simulink model "dynamicsquat"  (R2023a)
settings: Solver=VariableStepAuto  StartTime=0.0  StopTime=stoptimetotal  RelTol=1e-3
values from neighbouring files (symbols this model uses):
  battery = load('params/battery_Tattu.mat').battery    [runDetailedT18Model.m]
  IC = load('params/initialcond/IC_HoverAt30mOcto.mat').IC    [runDetailedT18Model.m]
  maxleashvelocity = 5    [runDetailedT18Model.m]
  Motor = load('params/KDE4213XF-360_performancedata.mat').Motor    [runDetailedT18Model.m]
  octomodel = load('params/TarotT18.mat').octomodel    [runDetailedT18Model.m]
  turbenabled = 0    [runDetailedT18Model.m]
  xref = xyzref(waypts,1)    [runDetailedT18Model.m]
  yref = xyzref(waypts,2)    [runDetailedT18Model.m]
  zref = xyzref(waypts,3)    [runDetailedT18Model.m]
undefined symbols (not defined in the file or in its folder): deg, DiscIntNeverNeededParam, F, Light, MIL, rad, s
libraries: aerolibconvert2 x2, shared6dof x1, aerolibwind2 x1
(part 2 of 2)

== system dynamicsquat/Motors/DC Motor 3/Mechanical part/torque and thrust calculation ==
  w angular speed : Inport
  Convert rad/s to rmp : Gain  Gain=60/(2*pi)
  "Propeller model " : MATLAB Function  TreatAsAtomicUnit=on
  torque : Outport  VectorParamsAs1DForOutWhenUnconnected=off
  thrusth : Outport  Port=2  VectorParamsAs1DForOutWhenUnconnected=off
  wires:
  Convert rad/s to rmp/1 -> "Propeller model "/1(rpm)
  w angular speed/1 -> Convert rad/s to rmp/1
  "Propeller model "/2(thrust) -> thrusth/1
  "Propeller model "/1(torque) -> torque/1

== system dynamicsquat/Motors/DC Motor 4/Mechanical part/torque and thrust calculation ==
  w angular speed : Inport
  Convert rad/s to rmp : Gain  Gain=60/(2*pi)
  "Propeller model " : MATLAB Function  TreatAsAtomicUnit=on
  torque : Outport  VectorParamsAs1DForOutWhenUnconnected=off
  thrusth : Outport  Port=2  VectorParamsAs1DForOutWhenUnconnected=off
  wires:
  "Propeller model "/1(torque) -> torque/1
  "Propeller model "/2(thrust) -> thrusth/1
  w angular speed/1 -> Convert rad/s to rmp/1
  Convert rad/s to rmp/1 -> "Propeller model "/1(rpm)

== system dynamicsquat/Motors/DC Motor 5/Mechanical part/torque and thrust calculation ==
  w angular speed : Inport
  Convert rad/s to rmp : Gain  Gain=60/(2*pi)
  "Propeller model " : MATLAB Function  TreatAsAtomicUnit=on
  torque : Outport  VectorParamsAs1DForOutWhenUnconnected=off
  thrusth : Outport  Port=2  VectorParamsAs1DForOutWhenUnconnected=off
  wires:
  Convert rad/s to rmp/1 -> "Propeller model "/1(rpm)
  w angular speed/1 -> Convert rad/s to rmp/1
  "Propeller model "/2(thrust) -> thrusth/1
  "Propeller model "/1(torque) -> torque/1

== system dynamicsquat/Motors/DC Motor 6/Mechanical part/torque and thrust calculation ==
  w angular speed : Inport
  Convert rad/s to rmp : Gain  Gain=60/(2*pi)
  "Propeller model " : MATLAB Function  TreatAsAtomicUnit=on
  torque : Outport  VectorParamsAs1DForOutWhenUnconnected=off
  thrusth : Outport  Port=2  VectorParamsAs1DForOutWhenUnconnected=off
  wires:
  "Propeller model "/1(torque) -> torque/1
  "Propeller model "/2(thrust) -> thrusth/1
  w angular speed/1 -> Convert rad/s to rmp/1
  Convert rad/s to rmp/1 -> "Propeller model "/1(rpm)

== system dynamicsquat/Motors/DC Motor 7/Mechanical part/torque and thrust calculation ==
  w angular speed : Inport
  Convert rad/s to rmp : Gain  Gain=60/(2*pi)
  "Propeller model " : MATLAB Function  TreatAsAtomicUnit=on
  torque : Outport  VectorParamsAs1DForOutWhenUnconnected=off
  thrusth : Outport  Port=2  VectorParamsAs1DForOutWhenUnconnected=off
  wires:
  Convert rad/s to rmp/1 -> "Propeller model "/1(rpm)
  w angular speed/1 -> Convert rad/s to rmp/1
  "Propeller model "/2(thrust) -> thrusth/1
  "Propeller model "/1(torque) -> torque/1

== system dynamicsquat/Motors/DC Motor 8/Mechanical part/torque and thrust calculation ==
  w angular speed : Inport
  Convert rad/s to rmp : Gain  Gain=60/(2*pi)
  "Propeller model " : MATLAB Function  TreatAsAtomicUnit=on
  torque : Outport  VectorParamsAs1DForOutWhenUnconnected=off
  thrusth : Outport  Port=2  VectorParamsAs1DForOutWhenUnconnected=off
  wires:
  "Propeller model "/1(torque) -> torque/1
  "Propeller model "/2(thrust) -> thrusth/1
  w angular speed/1 -> Convert rad/s to rmp/1
  Convert rad/s to rmp/1 -> "Propeller model "/1(rpm)

== matlab function dynamicsquat/Motors/DC Motor 8/Mechanical part/torque and thrust calculation/Propeller model  ==
  data: torque output; rpm input; thrust output
function [torque,thrust] = fcn(rpm)
%% Tarot model data

%coefficient of thrust, empirically derived
coef_t = 0.065;
%thrust = coef_t * density of air * velocity^2 * propeller diameter (m) ^4
%velocity in rev/sec, where  1 rev/sec = 1 rpm/60
thrust = coef_t*1.225*(rpm/60)^2*.47^4; % 18.5 inches ~ 0.47 m
% empirically derived
torque = (2.138e-08)*rpm^2 + (-1.279e-05)*rpm ;% (0.0216);

end

== matlab function dynamicsquat/Position//Velocity controllers/Velocity leashing ==
  data: refvelx input; ref_velx output; refvely input; refvelz input; The input; Phi input; Psi input; max_velocity input; ref_vely output; ref_velz output
function [ref_velx,ref_vely,ref_velz] = fcn(refvelx,refvely,refvelz,The,Phi,Psi,max_velocity)
%% convert to body frame velocity

% Earth/local/inertial to body frame DCM matrix (use transpose to transform to body frame from earth)
R_b_e = [cos(Psi)*cos(The) cos(Psi)*sin(The)*sin(Phi)-sin(Psi)*cos(Phi) cos(Psi)*sin(The)*cos(Phi)+sin(Psi)*sin(Phi);
       sin(Psi)*cos(The) sin(Psi)*sin(The)*sin(Phi)+cos(Psi)*cos(Phi) sin(Psi)*sin(The)*cos(Phi)-cos(Psi)*sin(Phi);
       -sin(The)         cos(The)*sin(Phi)                            cos(The)*cos(Phi)]; 

velinert=[refvelx,refvely,refvelz]';
velbody=R_b_e'*velinert;
velbody(3)=velinert(3);%z velocity measurement follows a different principle thus not affected by Euler angles

%% constraint max velocity 
ref_velocity=zeros(1,3);
if abs(norm(velbody)+ 1e-6)>max_velocity
    % preserve direction but constraint total velocity to max
    ref_velocity=(velbody/(norm(velbody)+ 1e-6))* max_velocity;
else
    ref_velocity=velbody;
end

 ref_velx=ref_velocity(1);
 ref_vely=ref_velocity(2);  
 ref_velz=ref_velocity(3);

== matlab function dynamicsquat/Power Consumption Calculation ==
  data: DC input; tot_mot_i output; Imot input
function tot_mot_i  = fcn(DC,Imot)
imot=zeros(8,1);
for i=1:length(DC)
    imot(i)=DC(i)*Imot(i);
end
tot_mot_i=sum(imot);
tot_mot_i=sum(Imot);
end

== matlab function dynamicsquat/Drag Force and Moment Calculation ==
  data: Vw_nom input; Fdrag output; Vw_turb input; Vb input; wb input; Mdrag output; Eul input; windspecs parameter
function [Fdrag,Mdrag]  = fcn(Vw_nom,Vw_turb,Vb,wb,Eul, windspecs)
%% Parameters 
% windspecs - airframe wind-related specs
% Vw_nom - nominal wind velocity in m/s in inertial frame
% Vw_turb - turbulence wind velocity in m/s in inertial frame
% Vb - linear velocity body frame
% wb - angular velocity body frame
% Eul - Euler angles inertial frame
model = windspecs;

% Z-Y-X rotation convention 
Phi = Eul(1);
The = Eul(2);
Psi = Eul(3);
R_b_e = [cos(Psi)*cos(The) cos(Psi)*sin(The)*sin(Phi)-sin(Psi)*cos(Phi) cos(Psi)*sin(The)*cos(Phi)+sin(Psi)*sin(Phi);
       sin(Psi)*cos(The) sin(Psi)*sin(The)*sin(Phi)+cos(Psi)*cos(Phi) sin(Psi)*sin(The)*cos(Phi)-cos(Psi)*sin(Phi);
       -sin(The)         cos(The)*sin(Phi)                            cos(The)*cos(Phi)]; % Rib
R_e_b = R_b_e'; % Rbi  

% 3-torque created by drag
p = wb(1);
q = wb(2);
r = wb(3);
Mdrag=(((-1/2)*model.rho*model.cd)*[model.Axy*p*abs(p)*model.lx model.Axy*q*abs(q)*model.ly 8*model.Ayz*r*abs(r)*model.lz])';

% Wind in the inertial frame

v_we=Vw_nom+Vw_turb; % wind velocity in m/s in inertial frame
v_wb=R_e_b*v_we; % wind velocity in m/s in body frame
v_a=v_wb+Vb; % apparent velocity resulting from wind and body

% 3-Drag force
Fdrag=(((-1/2)*model.rho*model.cd)*[model.Ayz*v_a(1)*abs(v_a(1)) model.Axz*v_a(2)*abs(v_a(2)) model.Axy*v_a(3)*abs(v_a(3))])';


end

== matlab function dynamicsquat/Adding attitude//ang vel noise ==
  data: u input; y output
function y = fcn(u)

y = zeros(6,1);
attnoisestd=0.0106;
angvelnoisestd=0.; 
% posnoisestd=0; 
% velnoisestd=0;
noiseatt=attnoisestd.*randn(3,1)*0;
noiseangvel=angvelnoisestd.*randn(3,1)*0;
noise=[noiseatt ;noiseangvel];
y = y + u + noise;

== matlab function dynamicsquat/Position//Velocity controllers/Position controllers ==
  data: reference input; ref_velx output double size=1; measurement input; ref_vely output double size=1; ref_velz output; errprev input size=[2 1]; errprev output; time input
function [ref_velx,ref_vely,ref_velz,errprev] = fcn(reference,measurement,errprev,time)
%% parameters
k_p=0.5;
k_d=0.05;%ki=;
dt=0.01; %controller frequency
% radius=2;

%% xyz separation

if time>0.12
    see=3.22;
end

%% z control signal calculation
kz_p=0.4;
errz = reference(3) - measurement(3);

% calculate desired velocity for z axis
err_pz = kz_p * errz; % offset based on minimum thrust to hover
ref_velz=err_pz;

%% xy control signal calculation
err = reference(1:2) - measurement(1:2);

%proximity check
% if abs(err(1))<radius
%     err(1)=0;
% end
% if abs(err(2))<radius
%     err(2)=0;
% end

% calculate desired velocity for xy axis
err_p = k_p * err;
% err_i = self.k_i * np.clip(
%     self.err_i + trapezoid((self.err, err), dx=self.dt, axis=0),
%     a_min=-self.max_err_i, a_max=self.max_err_i
% )
err_d = k_d * (err - errprev) / dt;
%direct velocity usage
ref_velxy=zeros(1,2);
ref_velx = err_p(1) ;%+ err_d2;%+ self.err_i ;
ref_vely = err_p(2) ;%+ err_d2;%+ self.err_i ;

% %% convert total vel to body-frame velocity
% velocity=zeros(1,3);
% velocity=[ref_velxy ref_velz];
% rot = [cos(yaw)   sin(yaw) 0; ...
%     -sin(yaw) cos(yaw) 0; ...
%     0           0      1];
% ref_velocity = rot * velocity; % velocity is a row vector [vx, vy, vz]
% 
% 
% % constraint max velocity 
% if abs(norm(ref_velocity)+ 1e-6)>max_velocity
%     % preserve direction but constraint total velocity to max
%     ref_velocity=(ref_velocity/norm(ref_velocity)+ 1e-6)* max_velocity;
% end
% 
%  ref_velx=ref_velocity(1);
%  ref_vely=ref_velocity(2);  
%  ref_velz=ref_velocity(3);  
% 
% errprev=err;

== matlab function dynamicsquat/arrival condition ==
  data: currentpos input; arrived output; dest input
function arrived = fcn(currentpos,dest)
result=norm(currentpos-dest);
if result<2 % less than one meter from the goal
    arrived=1;
else
    arrived=0;
end

== matlab function dynamicsquat/Adding position//velocity noise ==
  data: u input; y output
function y = fcn(u)

y = zeros(6,1);
posnoisestd=0.6; % 0.75 gives maximum and minimum of +-3 meters, 0.6 is +-2 meters
velnoisestd=0.02; % originally used 0.025
% posnoisestd=0; 
% velnoisestd=0;
noisepos=posnoisestd.*randn(3,1)*0;
noisevel=velnoisestd.*randn(3,1)*0;
noise=[noisepos ;noisevel];
y = y + u + noise;

y=round(y*100)/100;

== matlab function dynamicsquat/MATLAB Function ==
  data: x input; Wx output; y input; Wy output
function [Wx,Wy] = fcn(x,y)
% Interpolate wind speed components at aircraft position
coefs_u = [ 0.00000000e+00  1.61094414e-10 -7.37058611e-03 -1.48809651e-06...
    -3.68089481e-13 -7.95141020e-06  2.10701150e-17  9.01146727e-10...
    1.59724993e-17  6.10108129e-10  7.28957673e-14  8.49416234e-19...
    7.23116917e-13  4.75030720e-19  1.14705027e-12];
intercept_u = 10.362042657397877;

coefs_v = [ 0.00000000e+00 -2.00488263e-10  8.08528198e-03 -7.92842850e-07...
    4.03295347e-13  3.32875723e-06 -1.06781708e-17 -7.96012216e-11...
    -1.33310503e-17 -4.23514366e-09  7.95707308e-14 -4.36936906e-19...
    -5.13247109e-14 -4.72047951e-19 -1.17203841e-12];
intercept_v = 3.69631689881155;
degree = 4;

% Combine xs and ys into a single matrix of shape (n_samples, n_features)
features = [x, y];

    % Calculate the total number of polynomial features including the bias term
    totalFeatures = (degree + 1) * (degree + 2) / 2;
    
    [n_samples, ~] = size(features);
    
    % Preallocate polyFeatures matrix with zeros
    polyFeatures = zeros(n_samples, totalFeatures);
    
    % Fill in the bias (intercept) term
    polyFeatures(:, 1) = ones(n_samples, 1);
    
    % Index to keep track of the current column in polyFeatures
    currentColumn = 2;
    
    % Generate feature combinations and fill in polyFeatures
    for d = 1:degree
        for i = 0:d
            j = d - i;
            newFeature = (features(:,1).^i) .* (features(:,2).^j);
            polyFeatures(:, currentColumn) = newFeature;
            currentColumn = currentColumn + 1;
        end
    end

% Calculate the wind components by dot product, then add the intercept
Wx = (polyFeatures * coefs_u' + intercept_u)*0.5;
Wy = (polyFeatures * coefs_v' + intercept_v)*0.5;
end

== matlab function dynamicsquat/Motors/DC Motor 1/Mechanical part/torque and thrust calculation/Propeller model  ==
  data: torque output; rpm input; thrust output
function [torque,thrust] = fcn(rpm)
%% Tarot model data

%coefficient of thrust, empirically derived
coef_t = 0.065;
%thrust = coef_t * density of air * velocity^2 * propeller diameter (m) ^4
%velocity in rev/sec, where  1 rev/sec = 1 rpm/60
thrust = coef_t*1.225*(rpm/60)^2*.47^4; % 18.5 inches ~ 0.47 m
% empirically derived
torque = (2.138e-08)*rpm^2 + (-1.279e-05)*rpm ;% (0.0216);

end

== matlab function dynamicsquat/Forces and Moments Calculation ==
  data: w1 input; Fx output; w2 input; w3 input; w4 input; w5 input; w6 input; Fy output; Fz output; Mx output; My output; Mz output; w7 input; w8 input; Phi input; The input; Psi input; time input
function [Fx,Fy,Fz,Mx,My,Mz] = fcn(w1,w2,w3,w4,w5,w6,w7,w8,Phi,The,Psi,time)
octomodel.g=9.80;
octomodel.m_t=10.66;
octomodel.l=0.635;
% Phi,The,Psi, in rad
w  = [w1; w2; w3; w4;w5; w6; w7; w8];

if time>1.2
  see=1;
end

%% not used
%to fix numerical issues
%w=round(w,2);
% transform rpm to rad/s
%w=w./(60/(2*pi));

%% thrust generated by rotors

% Approach 1
% coef_t = 0.065;
%thrust = coef_t * density of air * velocity^2 * propeller diameter (m) ^4
%velocity in rev/sec, where  1 rev/sec = 1 rpm/60
%T = coef_t*1.225*((w./60).^2)*.47^4; % 18.5 inches ~ 0.47 m

% Approach 2
% thrust motor constant [Ns^2/rad^2]
b=9.8419e-05; % 
T = b.*((2*pi).*w./60).^2;

% total thrust generated by rotors
T_total=sum(T);
% T_total=round(T_total*100)/100;

%% Forces in the local frame 
R_b_e = [cos(Psi)*cos(The) cos(Psi)*sin(The)*sin(Phi)-sin(Psi)*cos(Phi) cos(Psi)*sin(The)*cos(Phi)+sin(Psi)*sin(Phi);
       sin(Psi)*cos(The) sin(Psi)*sin(The)*sin(Phi)+cos(Psi)*cos(Phi) sin(Psi)*sin(The)*cos(Phi)-cos(Psi)*sin(Phi);
       -sin(The)         cos(The)*sin(Phi)                            cos(The)*cos(Phi)]; % Rib

Ftot_b=R_b_e'*[0 ;0; -octomodel.m_t*octomodel.g]+[0; 0; T_total]; 
Ftot_b=round(Ftot_b*10)/10;
Fx=Ftot_b(1);Fy=Ftot_b(2);Fz=Ftot_b(3);

%% Moments in the local frame 
% moment of each rotor
% Approach 1
%M = (2.138e-08)*w.^2 + (-1.279e-05)*w ;

% Approach 2
% rotor drag constant [Nms^2/rad^2]
d=1.8503e-06; % 
M = d.*((2*pi).*w./60).^2;


% torque generated by rotors
%motor angles
angsm=cos(pi/8); % 22.5 
anglg=cos(3*pi/8); % 67.5

Mx=octomodel.l*(-T(1)*anglg -T(2)*angsm +T(3)*angsm +T(4)*anglg +T(5)*anglg ...
    +T(6)*angsm -T(7)*angsm -T(8)*anglg);%Tau_roll

My=octomodel.l*(-T(1)*angsm -T(2)*anglg -T(3)*anglg -T(4)*angsm +T(5)*angsm ...
    +T(6)*anglg +T(7)*anglg +T(8)*angsm);%Tau_theta

Mz= M(1) -M(2) +M(3) -M(4) +M(5) -M(6) +M(7) -M(8);%%Tau_yaw
end

== matlab function dynamicsquat/Motors/DC Motor 2/Mechanical part/torque and thrust calculation/Propeller model  ==
  data: torque output; rpm input; thrust output
function [torque,thrust] = fcn(rpm)
%% Tarot model data

%coefficient of thrust, empirically derived
coef_t = 0.065;
%thrust = coef_t * density of air * velocity^2 * propeller diameter (m) ^4
%velocity in rev/sec, where  1 rev/sec = 1 rpm/60
thrust = coef_t*1.225*(rpm/60)^2*.47^4; % 18.5 inches ~ 0.47 m
% empirically derived
torque = (2.138e-08)*rpm^2 + (-1.279e-05)*rpm ;% (0.0216);

end

== matlab function dynamicsquat/Motors/DC Motor 3/Mechanical part/torque and thrust calculation/Propeller model  ==
  data: torque output; rpm input; thrust output
function [torque,thrust] = fcn(rpm)
%% Tarot model data

%coefficient of thrust, empirically derived
coef_t = 0.065;
%thrust = coef_t * density of air * velocity^2 * propeller diameter (m) ^4
%velocity in rev/sec, where  1 rev/sec = 1 rpm/60
thrust = coef_t*1.225*(rpm/60)^2*.47^4; % 18.5 inches ~ 0.47 m
% empirically derived
torque = (2.138e-08)*rpm^2 + (-1.279e-05)*rpm ;% (0.0216);

end

== matlab function dynamicsquat/Motors/DC Motor 4/Mechanical part/torque and thrust calculation/Propeller model  ==
  data: torque output; rpm input; thrust output
function [torque,thrust] = fcn(rpm)
%% Tarot model data

%coefficient of thrust, empirically derived
coef_t = 0.065;
%thrust = coef_t * density of air * velocity^2 * propeller diameter (m) ^4
%velocity in rev/sec, where  1 rev/sec = 1 rpm/60
thrust = coef_t*1.225*(rpm/60)^2*.47^4; % 18.5 inches ~ 0.47 m
% empirically derived
torque = (2.138e-08)*rpm^2 + (-1.279e-05)*rpm ;% (0.0216);

end

== matlab function dynamicsquat/Motors/DC Motor 5/Mechanical part/torque and thrust calculation/Propeller model  ==
  data: torque output; rpm input; thrust output
function [torque,thrust] = fcn(rpm)
%% Tarot model data

%coefficient of thrust, empirically derived
coef_t = 0.065;
%thrust = coef_t * density of air * velocity^2 * propeller diameter (m) ^4
%velocity in rev/sec, where  1 rev/sec = 1 rpm/60
thrust = coef_t*1.225*(rpm/60)^2*.47^4; % 18.5 inches ~ 0.47 m
% empirically derived
torque = (2.138e-08)*rpm^2 + (-1.279e-05)*rpm ;% (0.0216);

end

== matlab function dynamicsquat/Motors/DC Motor 6/Mechanical part/torque and thrust calculation/Propeller model  ==
  data: torque output; rpm input; thrust output
function [torque,thrust] = fcn(rpm)
%% Tarot model data

%coefficient of thrust, empirically derived
coef_t = 0.065;
%thrust = coef_t * density of air * velocity^2 * propeller diameter (m) ^4
%velocity in rev/sec, where  1 rev/sec = 1 rpm/60
thrust = coef_t*1.225*(rpm/60)^2*.47^4; % 18.5 inches ~ 0.47 m
% empirically derived
torque = (2.138e-08)*rpm^2 + (-1.279e-05)*rpm ;% (0.0216);

end

== matlab function dynamicsquat/Motors/DC Motor 7/Mechanical part/torque and thrust calculation/Propeller model  ==
  data: torque output; rpm input; thrust output
function [torque,thrust] = fcn(rpm)
%% Tarot model data

%coefficient of thrust, empirically derived
coef_t = 0.065;
%thrust = coef_t * density of air * velocity^2 * propeller diameter (m) ^4
%velocity in rev/sec, where  1 rev/sec = 1 rpm/60
thrust = coef_t*1.225*(rpm/60)^2*.47^4; % 18.5 inches ~ 0.47 m
% empirically derived
torque = (2.138e-08)*rpm^2 + (-1.279e-05)*rpm ;% (0.0216);

end

== matlab function dynamicsquat/Control allocation ==
  data: Fx input; wref1 output; Fy input; Fz input; Troll input; Tpitch input; Tyaw input; wref2 output; wref3 output; wref4 output; wref5 output; wref6 output; wref7 output; wref8 output; Vbat input; DC output; time input
function [wref1,wref2,wref3,wref4,wref5,wref6,wref7,wref8,DC] = fcn(Fx,Fy,Fz,Troll,Tpitch,Tyaw,Vbat, time)
%% parameters 
%Maximum speed that the motors can reach in rad/s
Max_speed=670; %668.11
%Max total Thrust all motors can generate in N
Max_thrust=352; %351.451
%Max torque in each individual axis

% if time>4.9651
if time>1
    see=1;
end


% arm length - distances from the octorotor center of mass ...
%        to the center of mass of all its rotors are equal and denoted by l.
l=0.635;
% thrust motor constant [Ns^2/rad^2]
b=9.8419e-05; % 
% rotor drag constant [Nms^2/rad^2]
d=1.8503e-06; % 

%angles
angsm=cos(pi/8); % 22.5 
anglg=cos(3*pi/8); % 67.5

% control allocation matrix
A_f=[b b b b b b b b; ...
    -b*l*anglg -b*l*angsm b*l*angsm b*l*anglg b*l*anglg b*l*angsm -b*l*angsm -b*l*anglg; ...
    -b*l*angsm -b*l*anglg -b*l*anglg -b*l*angsm b*l*angsm b*l*anglg b*l*anglg b*l*angsm; ...
    d -d d -d d -d d -d];


% duty cycle initialization
DC=zeros(8,1);

%desired input
u_des=[Fz;Troll;Tpitch;Tyaw];

%control allocation
Omega_s=pinv(A_f)*u_des; %inverse of A_f is A_f\

% velocity checking
wref=zeros(8,1);
for i=1:length(Omega_s)
    if Omega_s(i)<0
        wref(i)=0;
    elseif Omega_s(i)>Max_speed^2
        wref(i)=Max_speed;
    else
        wref(i)=sqrt(Omega_s(i));
    end
end

wref=round(10*wref)/10;

%velocity assignment in V
DCfactor=0.001355; %original direct conversion multiply=0.0325; wref(i)=wref(i)*multiply;
Voltconversion=0.03249;% original 0.0325;



% "virtual" ESC 
for i=1:length(wref)
    % voltage saturation check
    if(wref(i)*DCfactor*Vbat > Vbat)
        wref(i)=Vbat;
        DC(i)=1;
    elseif(wref(i)*DCfactor*Vbat <=0)
        wref(i)=0.065;
        DC(i)=0.01;
    else
        DC(i)=wref(i)*DCfactor;
        %wref(i)=Vbat*DC(i); 
        wref(i)=wref(i)*Voltconversion;
    end
end

wref1=wref(1);
wref2=wref(2);
wref3=wref(3);
wref4=wref(4);
wref5=wref(5);
wref6=wref(6);
wref7=wref(7);
wref8=wref(8);


end
